simulink model "simulation"  (R2015a)
settings: Solver=ode45  StartTime=0.0  StopTime=10.0  RelTol=1e-3
libraries: simulink x1
settings Model: Creator=jonathan  LastModifiedBy=jonathan

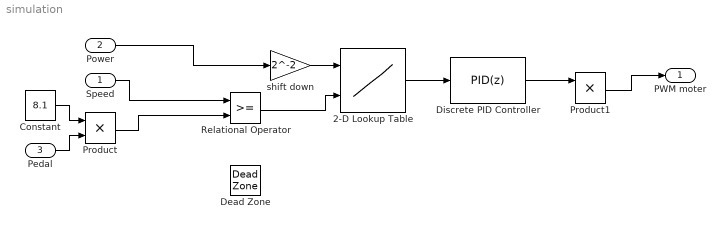
== system simulation ==
  Speed : Inport
  Power : Inport  Port=2
  Pedal : Inport  Port=3  OutDataTypeStr=boolean
  2-D Lookup Table : Lookup_n-D  BreakpointsForDimension1=[0:74]  BreakpointsForDimension2=[0:1]  Table=[6, 6, 13, 19, 26, 33, 39, 46, 53, 59, 66, 73, 79, 86, 93, 99, 106, 113, 114, 116, 118, 120, 122, 124, 126, 128, 130, 132, 134, 136, 138, 140, 142, 144, 146, 148, 149, 151, 153, 155, 157, 159, 161, 163, 165, 167, 170, 172, 175, 177, 180, 182, 184, 187, 189, 192, 194, 197, 199, 202, 204, 206, 209, 211, 214, 216, 219, 221, 223, 226, 228, 231, 233, 236, 238; 5, 25, 45, 51, 56, 62, 68, 73, 79, 84, 90, 96, 101, 107, 113, 119, 125, 131, 137, 143, 149, 155, 162, 168, 174, 180, 185, 191, 196, 202, 207, 213, 218, 224, 229, 235, 240, 244, 248, 252, 255, 255, 255, 255, 255, 255, 255, 255, 255, 255, 255, 255, 255, 255, 255, 255, 255, 255, 255, 255, 255, 255, 255, 255, 255, 255, 255, 255, 255, 255, 255, 255, 255, 255, 255]'  InternalRulePriority=Speed  RndMeth=Simplest  InputSameDT=on
  Constant : Constant  Value=8.1
  Dead Zone : DeadZone  LowerValue=-2  UpperValue=0  SaturateOnIntegerOverflow=on
  Discrete PID Controller : simulink/Continuous/PID Controller  Controller=PID  TimeDomain=Discrete-time  SampleTime=1  IntegratorMethod=Forward Euler  FilterMethod=Forward Euler  Form=Parallel  UseFilter=on  ControllerParametersSource=internal  P=1  I=1  D=0  N=100  InitialConditionSource=internal  InitialConditionForIntegrator=0  InitialConditionForFilter=0  ExternalReset=none  LimitOutput=off  UpperSaturationLimit=inf  LowerSaturationLimit=-inf  LinearizeAsGain=off  AntiWindupMode=none  Kb=1  TrackingMode=off  Kt=1  PParamMin=[]  PParamMax=[]  IParamMin=[]  IParamMax=[]  DParamMin=[]  DParamMax=[]  NParamMin=[]  NParamMax=[]  KbParamMin=[]  KbParamMax=[]  KtParamMin=[]  KtParamMax=[]  POutMin=[]  POutMax=[]  IOutMin=[]  IOutMax=[]  DOutMin=[]  DOutMax=[]  NOutMin=[]  NOutMax=[]  KbOutMin=[]  KbOutMax=[]  KtOutMin=[]  KtOutMax=[]  IntegratorOutMin=[]  IntegratorOutMax=[]  FilterOutMin=[]  FilterOutMax=[]  SumOutMin=[]  SumOutMax=[]  SumI1OutMin=[]  SumI1OutMax=[]  SumI2OutMin=[]  SumI2OutMax=[]  SumI3OutMin=[]  SumI3OutMax=[]  SumDOutMin=[]  SumDOutMax=[]  SaturationOutMin=[]  SaturationOutMax=[]  IntegratorContinuousStateAttributes=''  IntegratorStateMustResolveToSignalObject=off  IntegratorRTWStateStorageClass=Auto  FilterContinuousStateAttributes=''  FilterStateMustResolveToSignalObject=off  FilterRTWStateStorageClass=Auto  DifferentiatorICPrevScaledInput=0  DifferentiatorOutMin=[]  DifferentiatorOutMax=[]
  Product : Product
  Product1 : Product
  Relational Operator : RelationalOperator  OutDataTypeStr=boolean
  shift down : Gain  Gain=2^-2
  PWM moter : Outport
  wires:
  Relational Operator/1 -> 2-D Lookup Table/2
  2-D Lookup Table/1 -> Discrete PID Controller/1
  Constant/1 -> Product/1
  Product/1 -> Relational Operator/2
  Product1/1 -> PWM moter/1
  shift down/1 -> 2-D Lookup Table/1
  Power/1 -> shift down/1
  Speed/1 -> Relational Operator/1
  Discrete PID Controller/1 -> Product1/1
  Pedal/1 -> Product/2
